simulink model "M_NLdamper_plant"  (R2025b)
settings: Solver=daessc  StartTime=0.0  StopTime=t_slx_end  RelTol=1e-3  AbsTol=1e-3  EnableMultiTasking=on
undefined symbols (not defined in the file): DiscIntNeverNeededParam, l_length, mdta_cart, Ts, X, Y, Z
libraries: sm_lib x9, nesl_utility x5, cstblocks x2
settings Model: Creator=zxw20  LastModifiedBy=zxw20
settings SolverCC: AutoScaleAbsTol=off  AlgebraicLoopSolver=TrustRegion  MaxZcPerStep=1.0
settings DataIOCC: LimitDataPoints=on  MaxDataPoints=10000
settings OptimizationCC: ReuseModelBlockBuffer=off  LifeSpan=inf
settings DebuggingCC: UnconnectedInputMsg=warning  UnconnectedOutputMsg=warning  UnconnectedLineMsg=warning  AllowSymbolicDim=off  SubsystemReferenceDiagnosticForUnitTest=warning  SFUnexpectedBacktrackingDiag=warning  SFNoUnconditionalDefaultTransitionDiag=warning  SFExecutionAtInitializationDiag=none  ArithmeticOperatorsInVariantConditions=warning
settings ModelReferenceCC: EnableRefExpFcnMdlSchedulingChecks=on
settings SFSimCC: SimUseLocalCustomCode=off  CustomCodeUndefinedFunction=UseInterfaceOnly
settings RTWCC: RTWUseLocalCustomCode=off  GPUComputeCapability=3.5  DLArmComputeVersion=19.05
settings CodeAppCC: StateflowObjectComments=on
settings GRTTargetCC: TargetLangStandard=C89/C90 (ANSI)
settings ConfigComp: CovMetricSettings=dw  CovSaveCumulativeToWorkspaceVar=on  CovSaveSingleToWorkspaceVar=on  CovExternalEMLEnable=off  CovSFcnEnable=off
settings SimscapeCC: SimscapeLogType=all  SimscapeLogSimulationStatistics=on  SimscapeLogDataHistory=10000.0
settings ExplorerConfigSet: SimMechanicsOpenEditorOnUpdate=off

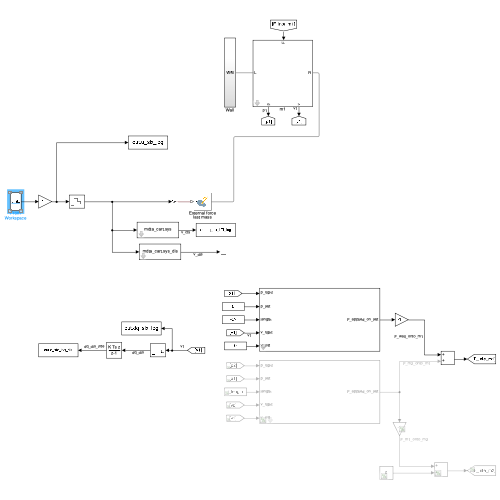
[thumbnail: Simulink's stored preview of the top-level diagram]
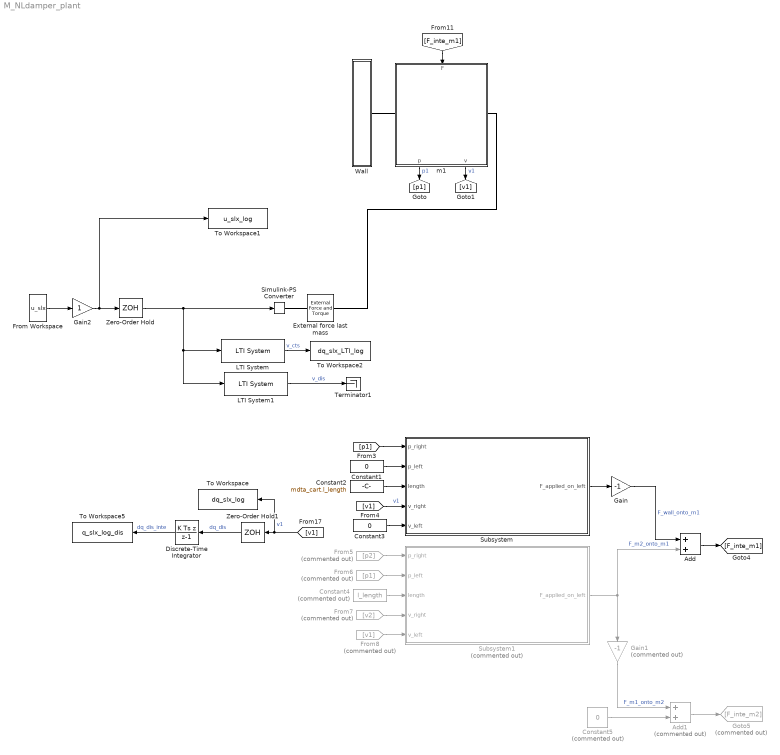
== system M_NLdamper_plant ==
  Add : Sum
  Add1 : Sum  Commented=on
  Constant1 : Constant  Value=0
  Constant2 : Constant  Value=mdta_cart.l_length
  Constant3 : Constant  Value=0
  Constant4 : Constant  Commented=on  Value=l_length
  Constant5 : Constant  Commented=on  Value=0
  Discrete-Time Integrator : DiscreteIntegrator  IntegratorMethod=Integration: Backward Euler  SampleTime=Ts  ICPrevOutput=DiscIntNeverNeededParam  ICPrevScaledInput=DiscIntNeverNeededParam
  External force last mass : sm_lib/Forces and Torques/External Force and Torque  EnableForceX=on  EnableForceY=off  EnableForceZ=off  EnableForce=off  ForceResolutionFrame=World  EnableTorqueX=off  EnableTorqueY=off  EnableTorqueZ=off  EnableTorque=off  TorqueResolutionFrame=AttachedFrame
  From Workspace : FromWorkspace  VariableName=u_slx  SampleTime=Ts  Interpolate=off  OutputAfterFinalValue=Holding final value
  From5 : From  Commented=on  GotoTag=p2
  From6 : From  Commented=on  GotoTag=p1
  From7 : From  Commented=on  GotoTag=v2
  From8 : From  Commented=on  GotoTag=v1
  Gain : Gain  Gain=-1
  Gain1 : Gain  Commented=on  Gain=-1
  Gain2 : Gain
  Goto5 : Goto  Commented=on  GotoTag=F_inte_m2
  LTI System : cstblocks/LTI System  sys=mdta_cart.sys  IC=[]  PadeOrder=0
  LTI System1 : cstblocks/LTI System  sys=mdta_cart.sys_dis  IC=[]  PadeOrder=0
  Simulink-PS Converter : nesl_utility/Simulink-PS Converter  PhysicalDomain=network_engine_domain  SubClassName=ps_input  LeftPortType=input  RightPortType=output  PseudoPeriodic=off  Frequencies=[]  NoiseDistribution=none  NoiseParameters=[]  Unit=1  AffineConversion=off  FilteringAndDerivatives=provide  SimscapeFilterOrder=1  InputFilterTimeConstant=0.001  UdotUserProvided=0
  Subsystem : Subsystem  mask{cart_spring_cst=mdta_cart.k(1), cart_L_damp_cst=mdta_cart.c(1), cart_NL_damp_cst=mdta_cart.c_NL(1)}
      mask DialogControl ParameterGroupVar Prompt: cart_para
  Subsystem1 : Subsystem  Commented=on  mask{cart_spring_cst=mdta_cart.k(1), cart_L_damp_cst=mdta_cart.c(1), cart_NL_damp_cst=mdta_cart.c_NL(1)}
      mask DialogControl ParameterGroupVar Prompt: cart_para
  Terminator1 : Terminator
  To Workspace : ToWorkspace  VariableName=dq_slx_log  SaveFormat=Structure With Time  SampleTime=Ts
  To Workspace1 : ToWorkspace  VariableName=u_slx_log  SaveFormat=Structure With Time  SampleTime=Ts
  To Workspace2 : ToWorkspace  VariableName=dq_slx_LTI_log  SaveFormat=Structure With Time  SampleTime=Ts
  To Workspace5 : ToWorkspace  VariableName=q_slx_log_dis  SaveFormat=Structure With Time  SampleTime=Ts
  Wall : Subsystem
  Zero-Order Hold : ZeroOrderHold  SampleTime=Ts
  Zero-Order Hold1 : ZeroOrderHold  SampleTime=Ts
  m1 : Subsystem  mask{cart_mass_kg=mdta_cart.m(1), spring_natural_length_m=mdta_cart.l_length}
      settings: PortSchema="{\"entries\":[{\"content\":{\"sides\":[{\"content\":{\"connectorIds\":[\"LConn1\"]},\"type\":\"ConnectorPlacement.EquallySpacedRectSide\",\"uuid\":\"4ce86df0-6398-4314-ae72-0c24d4f2584f\"},{\"content\":{\"connectorIds\":[\"RConn1\"],\"side\":\"RIGHT\"},\"type\":\"ConnectorPlacement.EquallySpacedRectSide\",\"uuid\":\"409d71ec-5ade-4475-9055-dc4a05333c88\"},{\"content\":{\"connectorIds\":[\"In1\"],\"side\":\"TOP\"},\"type\":\"ConnectorPlacement.EquallySpacedRectSide\",\"uuid\":\"5cf6242f-a793-405d-89da-ee6ed11b08b7\"},{\"content\":{\"connectorIds\":[\"Out1\",\"Out2\"],\"side\":\"BOTTOM\"},\"type\":\"ConnectorPlacement.EquallySpacedRectSide\",\"uuid\":\"38ef0f74-10f1-4eac-8fc8-477318099887\"}]},\"type\":\"ConnectorPlacement.EquallySpacedConnector\",\"uuid\":\"304aa765-4b2a-4ec8-93af-974d75c7ae4c\"}],\"packageUris\":[\"http://schema.mathworks.com/mf0/Connector/R2020b\"],\"version\":\"1.0\"}"
  wires:
  LTI System1/1 -> Terminator1/1  "v_dis"
  Constant1/1 -> Subsystem/2(p_left)
  [p1] -> Subsystem/1(p_right)
  Constant2/1 -> Subsystem/3(length)
  [v1] -> Subsystem/4(v_right)  "v1"
  Constant3/1 -> Subsystem/5(v_left)
  Subsystem/1(F_applied_on_left) -> Gain/1
  Gain/1 -> Add/1  "F_wall_onto_m1"
  From5/1 -> Subsystem1/1(p_right)
  From6/1 -> Subsystem1/2(p_left)
  Constant4/1 -> Subsystem1/3(length)
  From7/1 -> Subsystem1/4(v_right)
  From8/1 -> Subsystem1/5(v_left)
  Subsystem1/1(F_applied_on_left) -> Add/2, Gain1/1  "F_m2_onto_m1"
  Add/1 -> [F_inte_m1]
  Gain1/1 -> Add1/1  "F_m1_onto_m2"
  Constant5/1 -> Add1/2
  Add1/1 -> Goto5/1
  [F_inte_m1] -> m1/1(F)
  m1/1(p) -> [p1]  "p1"
  m1/2(v) -> [v1]  "v1"
  Zero-Order Hold/1 -> Simulink-PS Converter/1, LTI System/1, LTI System1/1
  Discrete-Time Integrator/1 -> To Workspace5/1  "dq_dis_inte"
  Zero-Order Hold1/1 -> Discrete-Time Integrator/1  "dq_dis"
  [v1] -> To Workspace/1, Zero-Order Hold1/1  "v1"
  LTI System/1 -> To Workspace2/1  "v_cts"
  Gain2/1 -> To Workspace1/1, Zero-Order Hold/1
  From Workspace/1 -> Gain2/1
  connections:
  m1/RConn1 -- External force last mass/RConn1
  m1/LConn1 -- Wall/RConn1
  Simulink-PS Converter/RConn1 -- External force last mass/LConn1

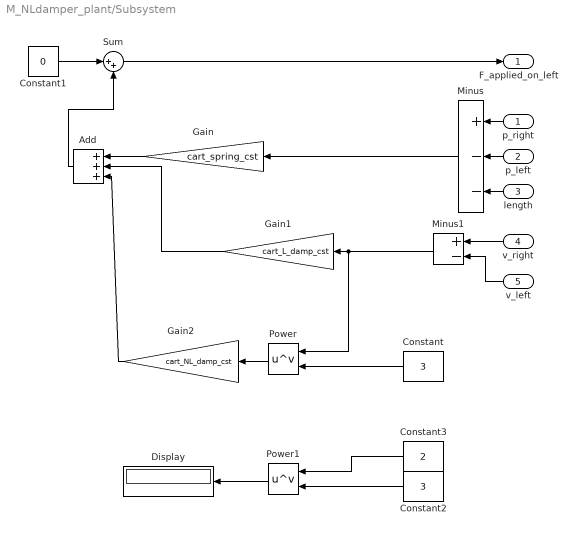
== system M_NLdamper_plant/Subsystem ==
  p_right : Inport
  p_left : Inport  Port=2
  length : Inport  Port=3
  v_right : Inport  Port=4
  v_left : Inport  Port=5
  Add : Sum  Inputs=+++
  Constant : Constant  Value=3
  Constant1 : Constant  Value=0
  Constant2 : Constant  Value=3
  Constant3 : Constant  Value=2
  Display : Display
  Gain : Gain  Gain=cart_spring_cst
  Gain1 : Gain  Gain=cart_L_damp_cst
  Gain2 : Gain  Gain=cart_NL_damp_cst
  Minus : Sum  Inputs=+--
  Minus1 : Sum  Inputs=+-
  Power : Math  Operator=pow
  Power1 : Math  Operator=pow
  Sum : Sum  Inputs=|++
  F_applied_on_left : Outport
  wires:
  length/1 -> Minus/3
  v_right/1 -> Minus1/1
  p_left/1 -> Minus/2
  Constant1/1 -> Sum/1
  Gain/1 -> Add/1
  Gain1/1 -> Add/2
  Minus/1 -> Gain/1
  Sum/1 -> F_applied_on_left/1
  p_right/1 -> Minus/1
  v_left/1 -> Minus1/2
  Minus1/1 -> Power/1, Gain1/1
  Add/1 -> Sum/2
  Constant/1 -> Power/2
  Power/1 -> Gain2/1
  Gain2/1 -> Add/3
  Power1/1 -> Display/1
  Constant2/1 -> Power1/2
  Constant3/1 -> Power1/1

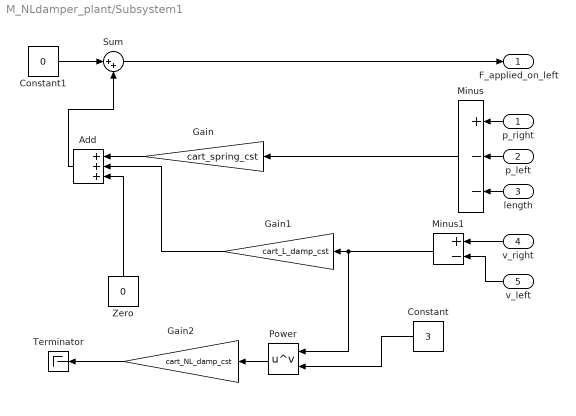
== system M_NLdamper_plant/Subsystem1 ==
  p_right : Inport
  p_left : Inport  Port=2
  length : Inport  Port=3
  v_right : Inport  Port=4
  v_left : Inport  Port=5
  Add : Sum  Inputs=+++
  Constant : Constant  Value=3
  Constant1 : Constant  Value=0
  Gain : Gain  Gain=cart_spring_cst
  Gain1 : Gain  Gain=cart_L_damp_cst
  Gain2 : Gain  Gain=cart_NL_damp_cst
  Minus : Sum  Inputs=+--
  Minus1 : Sum  Inputs=+-
  Power : Math  Operator=pow
  Sum : Sum  Inputs=|++
  Terminator : Terminator
  Zero : Constant  Value=0  OutDataTypeStr=Inherit: Inherit via back propagation
  F_applied_on_left : Outport
  wires:
  length/1 -> Minus/3
  v_right/1 -> Minus1/1
  p_left/1 -> Minus/2
  Constant1/1 -> Sum/1
  Gain/1 -> Add/1
  Gain1/1 -> Add/2
  Minus/1 -> Gain/1
  Sum/1 -> F_applied_on_left/1
  p_right/1 -> Minus/1
  v_left/1 -> Minus1/2
  Minus1/1 -> Power/1, Gain1/1
  Add/1 -> Sum/2
  Constant/1 -> Power/2
  Power/1 -> Gain2/1
  Gain2/1 -> Terminator/1
  Zero/1 -> Add/3

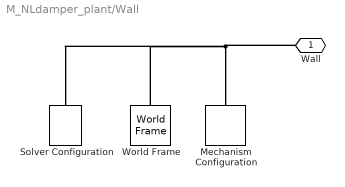
== system M_NLdamper_plant/Wall ==
  Mechanism Configuration : sm_lib/Utilities/Mechanism Configuration  UniformGravity=Constant  GravityVector=[0 0 0]  GravityVectorUnits=m/s^2  LinearizationDelta=0.001  JointModeTransitionNonlinearIterations=2
  Solver Configuration : nesl_utility/Solver Configuration  PhysicalDomain=network_engine_domain  SubClassName=solver  LeftPortType=input  RightPortType=generic  Tones=[]  Harmonics=[]  SimulateNoise=off  Profile=off  UseLocalSampling=off  EnableSwitchedLinearOptims=on  FrequencyDomain=off  UseCCode=off  RelTol=0.001  AbsTol=1e-06  MinStep=1e-09  ToWorkspace=off  RevertToSquareIcSolve=off  NumHomotopyIterations=100  PhasorMode=off  PhasorModeNumHarmonics=1  ConsistencySolver=NEWTON_XTOL_AFTER_FTOL  IndexReductionMethod=DerivativeReplacement  DoDC=off  ResidualTolerance=1e-09  ConsistencyTolSource=GLOBAL  ConsistencyAbsTol=0.001  ConsistencyRelTol=0.001  ConsistencyTolFactor=0.001  UseLocalSolver=off  LocalSolverChoice=NE_BACKWARD_EULER_ADVANCER  ResolveIndetEquations=on  FunctionEvalNumThread=1  LocalSolverSampleTime=0.001  DoFixedCost=off  MaxNonlinIter=3  MaxModeIter=2  ComputeImpulses=off  ImpulseIterations=2  LinearAlgebra=Sparse  LinearAlgebraNumThread=0  EquationFormulation=NE_TIME_EF  DelaysMemoryBudget=1024  AutomaticFiltering=on  FilteringTimeConstant=0.001  PartitionStorageMethod=AS_NEEDED  PartitionMemoryBudget=1024  PartitionMethod=FAST  MultibodyUseLocalSolver=off  MultibodyLocalSolverChoice=ODE1  MultibodyLocalSolverSampleTime=0.001
  World Frame : sm_lib/Frames and Transforms/World Frame
  Wall : PMIOPort  Side=Right
  connections:
  World Frame/RConn1 -- Solver Configuration/RConn1 -- Wall/RConn1 -- Mechanism Configuration/RConn1

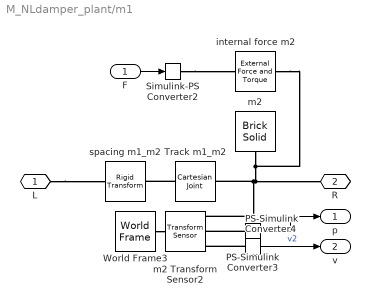
== system M_NLdamper_plant/m1 ==
  F : Inport
  PS-Simulink Converter3 : nesl_utility/PS-Simulink Converter  PhysicalDomain=network_engine_domain  SubClassName=ps_output  LeftPortType=input  RightPortType=output  PseudoPeriodic=off  Frequencies=[]  VectorFormat=inherit  Unit=inherit  AffineConversion=off
  PS-Simulink Converter4 : nesl_utility/PS-Simulink Converter  PhysicalDomain=network_engine_domain  SubClassName=ps_output  LeftPortType=input  RightPortType=output  PseudoPeriodic=off  Frequencies=[]  VectorFormat=inherit  Unit=inherit  AffineConversion=off
  Simulink-PS Converter2 : nesl_utility/Simulink-PS Converter  PhysicalDomain=network_engine_domain  SubClassName=ps_input  LeftPortType=input  RightPortType=output  PseudoPeriodic=off  Frequencies=[]  NoiseDistribution=none  NoiseParameters=[]  Unit=1  AffineConversion=off  FilteringAndDerivatives=provide  SimscapeFilterOrder=1  InputFilterTimeConstant=0.001  UdotUserProvided=0
  Track m1_m2 : sm_lib/Joints/Cartesian Joint  JointMode=Normal  CompositeWrenchDir=FollowerOnBase  CompositeWrenchFrame=BaseFrame  SenseConstraintForce=off  SenseConstraintTorque=off  SenseTotalForce=off  SenseTotalTorque=off  PxPositionTargetSpecify=off  PxPositionTargetPriority=High  PxPositionTargetValue=0  PxPositionTargetValueUnits=m  PxVelocityTargetSpecify=off  PxVelocityTargetPriority=High  PxVelocityTargetValue=0  PxVelocityTargetValueUnits=m/s  PxEquilibriumPosition=0  PxEquilibriumPositionUnits=m  PxSpringStiffness=0  PxSpringStiffnessUnits=N/m  PxDampingCoefficient=0  PxDampingCoefficientUnits=N/(m/s)  PxLowerLimitSpecify=off  PxLowerLimitBound=-1  PxLowerLimitBoundUnits=m  PxLowerLimitStiffness=1e6  PxLowerLimitStiffnessUnits=N/m  PxLowerLimitDamping=1e3  PxLowerLimitDampingUnits=N/(m/s)  PxLowerLimitTransitionRegionWidth=1e-4  PxLowerLimitTransitionRegionWidthUnits=m  PxUpperLimitSpecify=off  PxUpperLimitBound=1  PxUpperLimitBoundUnits=m  PxUpperLimitStiffness=1e6  PxUpperLimitStiffnessUnits=N/m  PxUpperLimitDamping=1e3  PxUpperLimitDampingUnits=N/(m/s)  PxUpperLimitTransitionRegionWidth=1e-4  PxUpperLimitTransitionRegionWidthUnits=m  PxTorqueActuationMode=NoTorque  PxMotionActuationMode=ComputedMotion  PxSensePosition=off  PxSenseVelocity=off  PxSenseAcceleration=off  PxSenseTorqueForce=off  PxSenseLowerLimitTorqueForce=off  PxSenseUpperLimitTorqueForce=off  PyPositionTargetSpecify=off  PyPositionTargetPriority=High  PyPositionTargetValue=0  PyPositionTargetValueUnits=m  PyVelocityTargetSpecify=off  PyVelocityTargetPriority=High  PyVelocityTargetValue=0  PyVelocityTargetValueUnits=m/s  PyEquilibriumPosition=0  PyEquilibriumPositionUnits=m  PySpringStiffness=0  PySpringStiffnessUnits=N/m  PyDampingCoefficient=0  PyDampingCoefficientUnits=N/(m/s)  PyLowerLimitSpecify=off  PyLowerLimitBound=-1  PyLowerLimitBoundUnits=m  PyLowerLimitStiffness=1e6  PyLowerLimitStiffnessUnits=N/m  PyLowerLimitDamping=1e3  PyLowerLimitDampingUnits=N/(m/s)  PyLowerLimitTransitionRegionWidth=1e-4  PyLowerLimitTransitionRegionWidthUnits=m  PyUpperLimitSpecify=off  PyUpperLimitBound=1  PyUpperLimitBoundUnits=m  PyUpperLimitStiffness=1e6  PyUpperLimitStiffnessUnits=N/m  PyUpperLimitDamping=1e3  PyUpperLimitDampingUnits=N/(m/s)  PyUpperLimitTransitionRegionWidth=1e-4  PyUpperLimitTransitionRegionWidthUnits=m  PyTorqueActuationMode=NoTorque  PyMotionActuationMode=ComputedMotion  PySensePosition=off  PySenseVelocity=off  PySenseAcceleration=off  PySenseTorqueForce=off  PySenseLowerLimitTorqueForce=off  PySenseUpperLimitTorqueForce=off  PzPositionTargetSpecify=off  PzPositionTargetPriority=High  PzPositionTargetValue=0  PzPositionTargetValueUnits=m  PzVelocityTargetSpecify=off  PzVelocityTargetPriority=High  PzVelocityTargetValue=0  PzVelocityTargetValueUnits=m/s  PzEquilibriumPosition=0  PzEquilibriumPositionUnits=m  PzSpringStiffness=0  PzSpringStiffnessUnits=N/m  PzDampingCoefficient=0  PzDampingCoefficientUnits=N/(m/s)  PzLowerLimitSpecify=off  PzLowerLimitBound=-1  PzLowerLimitBoundUnits=m  PzLowerLimitStiffness=1e6  PzLowerLimitStiffnessUnits=N/m  PzLowerLimitDamping=1e3  PzLowerLimitDampingUnits=N/(m/s)  PzLowerLimitTransitionRegionWidth=1e-4  PzLowerLimitTransitionRegionWidthUnits=m  PzUpperLimitSpecify=off  PzUpperLimitBound=1  PzUpperLimitBoundUnits=m  PzUpperLimitStiffness=1e6  PzUpperLimitStiffnessUnits=N/m  PzUpperLimitDamping=1e3  PzUpperLimitDampingUnits=N/(m/s)  PzUpperLimitTransitionRegionWidth=1e-4  PzUpperLimitTransitionRegionWidthUnits=m  PzTorqueActuationMode=NoTorque  PzMotionActuationMode=ComputedMotion  PzSensePosition=off  PzSenseVelocity=off  PzSenseAcceleration=off  PzSenseTorqueForce=off  PzSenseLowerLimitTorqueForce=off  PzSenseUpperLimitTorqueForce=off
  World Frame3 : sm_lib/Frames and Transforms/World Frame
  internal force m2 : sm_lib/Forces and Torques/External Force and Torque  EnableForceX=on  EnableForceY=off  EnableForceZ=off  EnableForce=off  ForceResolutionFrame=World  EnableTorqueX=off  EnableTorqueY=off  EnableTorqueZ=off  EnableTorque=off  TorqueResolutionFrame=AttachedFrame
  m2 : sm_lib/Body Elements/Brick Solid  BrickDimensions=[0.1 0.03 0.1]  BrickDimensionsUnits=m  ExportEntireGeometry=off  InertiaType=PointMass  BasedOnType=Density  Density=1000  DensityUnits=kg/m^3  Mass=cart_mass_kg  MassUnits=kg  CenterOfMass=[0 0 0]  CenterOfMassUnits=m  MomentsOfInertia=[1 1 1]  MomentsOfInertiaUnits=kg*m^2  ProductsOfInertia=[0 0 0]  ProductsOfInertiaUnits=kg*m^2  GraphicType=FromGeometry  MarkerShape=Sphere  MarkerSize=10  GraphicVisPropType=SimpleVisualProperties  GraphicDiffuseColor=[0.4549 0.5725 0.498]  GraphicOpacity=0.5  GraphicSpecularColor=[0.5 0.5 0.5 1.0]  GraphicAmbientColor=[0.15 0.15 0.15 1.0]  GraphicEmissiveColor=[0.0 0.0 0.0 1.0]  GraphicShininess=75  DoExposeReferenceFrame=on  SerializedFrames=<Frames/>
  m2 Transform Sensor2 : sm_lib/Frames and Transforms/Transform Sensor  MeasurementFrame=World  RotationSequence=XYX  SenseAngle=off  SenseAxis=off  SenseQ=off  SenseR=off  SenseRotationSequence=off  SenseOmegaX=off  SenseOmegaY=off  SenseOmegaZ=off  SenseOmega=off  SenseQDot=off  SenseRDot=off  SenseRotationSequenceDot=off  SenseAlphaX=off  SenseAlphaY=off  SenseAlphaZ=off  SenseAlpha=off  SenseQDDot=off  SenseRDDot=off  SenseX=on  SenseY=off  SenseZ=off  SenseXYZ=off  SenseRad=off  SenseAzim=off  SenseDist=off  SenseInc=off  SenseXDot=on  SenseYDot=off  SenseZDot=off  SenseXYZDot=off  SenseRadDot=off  SenseAzimDot=off  SenseDistDot=off  SenseIncDot=off  SenseXDDot=off  SenseYDDot=off  SenseZDDot=off  SenseXYZDDot=off  SenseRadDDot=off  SenseAzimDDot=off  SenseDistDDot=off  SenseIncDDot=off
  spacing m1_m2 : sm_lib/Frames and Transforms/Rigid Transform  RotationMethod=None  FollAlignAxisA=+X  BaseAlignAxisA=+Y  FollAlignAxisB=+Y  BaseAlignAxisB=+Z  RotationStandardAxis=+Z  RotationAngle=0  RotationAngleUnits=deg  RotationArbitraryAxis=[0 0 1]  RotationSequenceAxes=FollowerAxes  RotationSequence=XYX  RotationSequenceAngles=[0 0 0]  RotationSequenceAnglesUnits=deg  RotationMatrix=[1 0 0;0 1 0;0 0 1]  Quaternion=[1 0 0 0]  TranslationMethod=StandardAxis  TranslationCartesianOffset=[0 0 0]  TranslationCartesianOffsetUnits=m  TranslationStandardAxis=+X  TranslationStandardOffset=spring_natural_length_m  TranslationStandardOffsetUnits=m  TranslationROffset=0  TranslationROffsetUnits=m  TranslationThetaOffset=0  TranslationThetaOffsetUnits=deg  TranslationZOffset=0  TranslationZOffsetUnits=m
  L : PMIOPort  Side=Left
  R : PMIOPort  Port=2  Side=Right
  p : Outport
  v : Outport  Port=2
  wires:
  PS-Simulink Converter4/1 -> v/1  "v2"
  PS-Simulink Converter3/1 -> p/1
  F/1 -> Simulink-PS Converter2/1
  connections:
  PS-Simulink Converter3/LConn1 -- m2 Transform Sensor2/RConn2
  Track m1_m2/LConn1 -- spacing m1_m2/RConn1
  PS-Simulink Converter4/LConn1 -- m2 Transform Sensor2/RConn3
  World Frame3/RConn1 -- m2 Transform Sensor2/LConn1
  L/RConn1 -- spacing m1_m2/LConn1
  internal force m2/RConn1 -- m2/RConn1 -- Track m1_m2/RConn1 -- m2 Transform Sensor2/RConn1 -- R/RConn1
  Simulink-PS Converter2/RConn1 -- internal force m2/LConn1
